simulink model "One_Shot_Simulation"  (R2018b)
settings: Solver=VariableStepAuto  StartTime=0.0  StopTime=5  RelTol=1e-3
libraries: simulink x1, truetime x1
settings Model: Creator=ortegafausto  LastModifiedBy=of
settings SFSimCC: SimUseLocalCustomCode=off
settings RTWCC: RTWUseLocalCustomCode=off
settings CodeAppCC: StateflowObjectComments=on
settings SimscapeCC: SimscapeNormalizeSystem=off

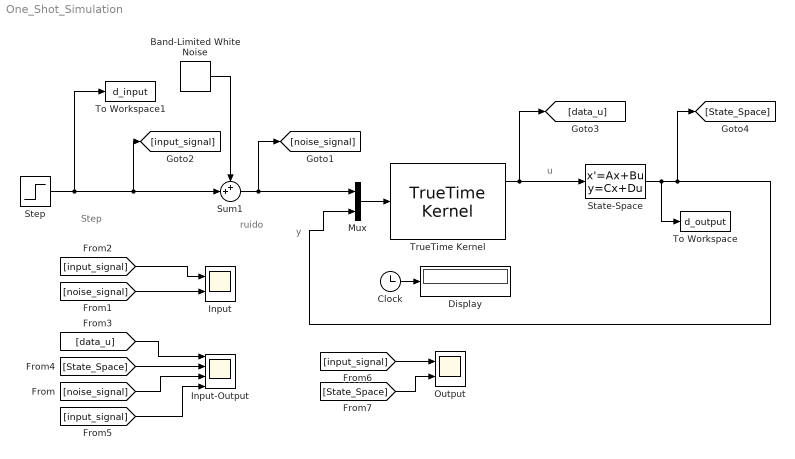
== system One_Shot_Simulation ==
  note: u
  note: Step
  note: ruido
  note: y
  Band-Limited White Noise : simulink/Sources/Band-Limited White Noise  Cov=[0.00005]  Ts=0.01  seed=[23341]
  Clock : Clock
  Display : Display
  "Input " : Scope  NumInputPorts=2
  "Input-Output " : Scope  NumInputPorts=4
  Mux : Mux  Inputs=2
  "Output " : Scope  NumInputPorts=2
  State-Space : StateSpace  A=[0 1;-918 -90.9]  B=[0; 918.27]  C=[1 0]  D=0  InitialCondition=0
  Step : Step  After=2.4  SampleTime=0
  Sum1 : Sum  Inputs=++|
  To Workspace : ToWorkspace  VariableName=d_output  SampleTime=-1
  To Workspace1 : ToWorkspace  VariableName=d_input  SampleTime=-1
  TrueTime Kernel : truetime/TrueTime Kernel  sfun=one_shot_init  args=[]  ninputsoutputs=[2 1]  ntriggers=0  trigtype=falling  nwnodenbr=[]  clockoffsetdrift=[0 0]  schedoutput=on  battery=off  poweroutput=off
  wires:
  Clock/1 -> Display/1
  Mux/1 -> TrueTime Kernel/1
  TrueTime Kernel/1 -> [data_u], State-Space/1
  Step/1 -> To Workspace1/1, [input_signal], Sum1/2
  State-Space/1 -> To Workspace/1, [State_Space], Mux/2
  Band-Limited White Noise/1 -> Sum1/1
  [noise_signal] -> "Input-Output "/3
  [noise_signal] -> "Input "/2
  [input_signal] -> "Input "/1
  [data_u] -> "Input-Output "/1
  [State_Space] -> "Input-Output "/2
  [input_signal] -> "Input-Output "/4
  [input_signal] -> "Output "/1
  [State_Space] -> "Output "/2
  Sum1/1 -> Mux/1, [noise_signal]
